simulink model "final_project"  (R2022a)
settings: Solver=VariableStepAuto  StartTime=0.0  StopTime=12  RelTol=1e-3
undefined symbols (not defined in the file or in its folder): C, vinit, Vref
libraries: SignalEditorBlockLib x2
settings Model: Creator=risha  LastModifiedBy=risha

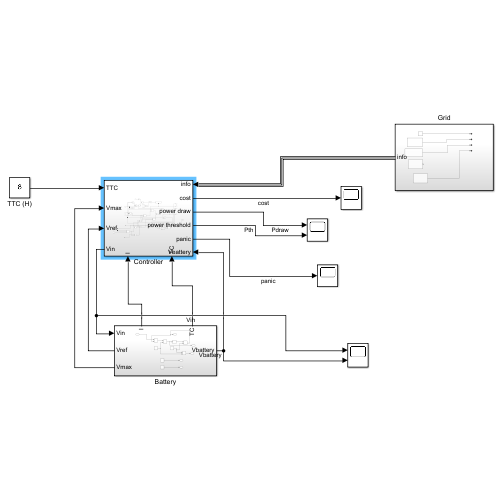
[thumbnail: Simulink's stored preview of the top-level diagram]
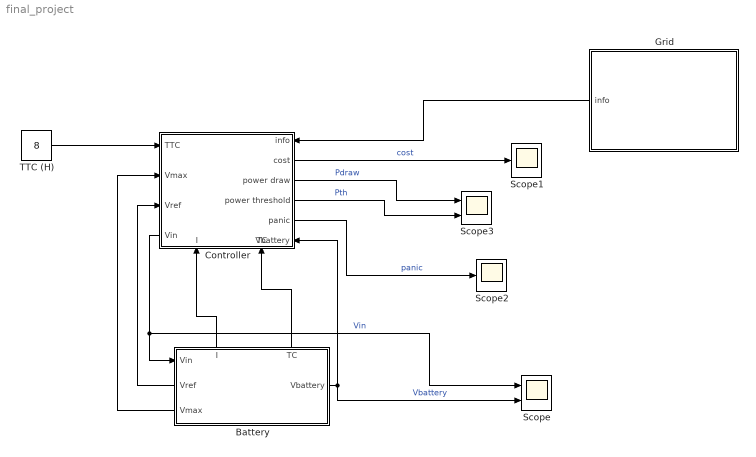
== system final_project ==
  Battery : Subsystem
      settings: PortSchema="{\"entries\":[{\"content\":{\"sides\":[{\"content\":{\"connectorIds\":[\"In1\",\"Out4\",\"Out5\"]},\"type\":\"ConnectorPlacement.EquallySpacedRectSide\",\"uuid\":\"c26d1ca6-d5c6-41a9-a1a0-e3693243df6e\"},{\"content\":{\"connectorIds\":[\"Out1\"],\"side\":\"RIGHT\"},\"type\":\"ConnectorPlacement.EquallySpacedRectSide\",\"uuid\":\"035a91c5-644a-4a3c-8d91-d0006be2b843\"},{\"content\":{\"connectorIds\":[\"Out2\",\"Out3\"],\"side\":\"TOP\"},\"type\":\"ConnectorPlacement.EquallySpacedRectSide\",\"uuid\":\"240e333e-0db7-4e7b-b69e-e92fd9d26be7\"}]},\"type\":\"ConnectorPlacement.EquallySpacedConnector\",\"uuid\":\"79b69b51-48a7-4588-8c16-b604fd62fdea\"}],\"packageUris\":[\"http://schema.mathworks.com/mf0/Connector/R2020b\"],\"version\":\"1.0\"}"
  Controller : Subsystem
      settings: PortSchema="{\"entries\":[{\"content\":{\"sides\":[{\"content\":{\"connectorIds\":[\"In1\",\"In2\",\"In3\",\"Out5\"]},\"type\":\"ConnectorPlacement.EquallySpacedRectSide\",\"uuid\":\"c26d1ca6-d5c6-41a9-a1a0-e3693243df6e\"},{\"content\":{\"connectorIds\":[\"In6\",\"Out1\",\"Out2\",\"Out3\",\"Out4\",\"In7\"],\"side\":\"RIGHT\"},\"type\":\"ConnectorPlacement.EquallySpacedRectSide\",\"uuid\":\"035a91c5-644a-4a3c-8d91-d0006be2b843\"},{\"content\":{\"connectorIds\":[],\"side\":\"TOP\"},\"type\":\"ConnectorPlacement.EquallySpacedRectSide\",\"uuid\":\"240e333e-0db7-4e7b-b69e-e92fd9d26be7\"},{\"content\":{\"connectorIds\":[\"In4\",\"In5\"],\"side\":\"BOTTOM\"},\"type\":\"ConnectorPlacement.EquallySpacedRectSide\",\"uuid\":\"1901438f-64d2-437a-91ec-20947983ea35\"}]},\"type\":\"ConnectorPlacement.EquallySpacedConnector\",\"uuid\":\"79b69b51-48a7-4588-8c16-b604fd62fdea\"}],\"packageUris\":[\"http://schema.mathworks.com/mf0/Connector/R2020b\"],\"version\":\"1.0\"}"
  Grid : Subsystem
  Scope : Scope  NumInputPorts=2
  Scope1 : Scope
  Scope2 : Scope
  Scope3 : Scope  NumInputPorts=2
  TTC (H) : Constant  Value=8
  wires:
  Battery/1(Vbattery) -> Scope/2, Controller/7(Vbattery)  "Vbattery"
  Controller/5(Vin) -> Scope/1, Battery/1(Vin)  "Vin"
  Grid/1(info) -> Controller/6(info)
  TTC (H)/1 -> Controller/1(TTC)
  Battery/4(Vref) -> Controller/3(Vref)
  Controller/1(cost) -> Scope1/1  "cost"
  Battery/3(TC) -> Controller/5(TC)
  Battery/5(Vmax) -> Controller/2(Vmax)
  Battery/2(I) -> Controller/4(I)
  Controller/4(panic) -> Scope2/1  "panic"
  Controller/2(power draw) -> Scope3/1  "Pdraw"
  Controller/3(power threshold) -> Scope3/2  "Pth"

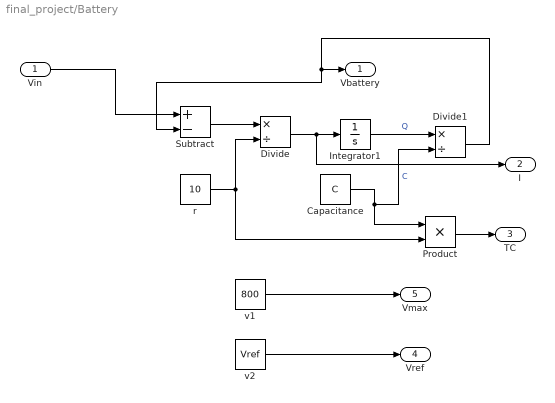
== system final_project/Battery ==
  Vin : Inport
  Capacitance : Constant  Value=C
  Divide : Product  Inputs=*/
  Divide1 : Product  Inputs=*/
  Integrator1 : Integrator  InitialCondition=C*vinit
  Product : Product
  Subtract : Sum  Inputs=+-
  r : Constant  Value=10
  v1 : Constant  Value=800
  v2 : Constant  Value=Vref
  Vbattery : Outport
  I : Outport  Port=2
  TC : Outport  Port=3
  Vref : Outport  Port=4
  Vmax : Outport  Port=5
  wires:
  Vin/1 -> Subtract/1
  Subtract/1 -> Divide/1
  r/1 -> Divide/2, Product/2
  Divide/1 -> I/1, Integrator1/1
  Integrator1/1 -> Divide1/1  "Q"
  Capacitance/1 -> Product/1, Divide1/2  "C"
  Divide1/1 -> Subtract/2, Vbattery/1
  v1/1 -> Vmax/1
  v2/1 -> Vref/1
  Product/1 -> TC/1

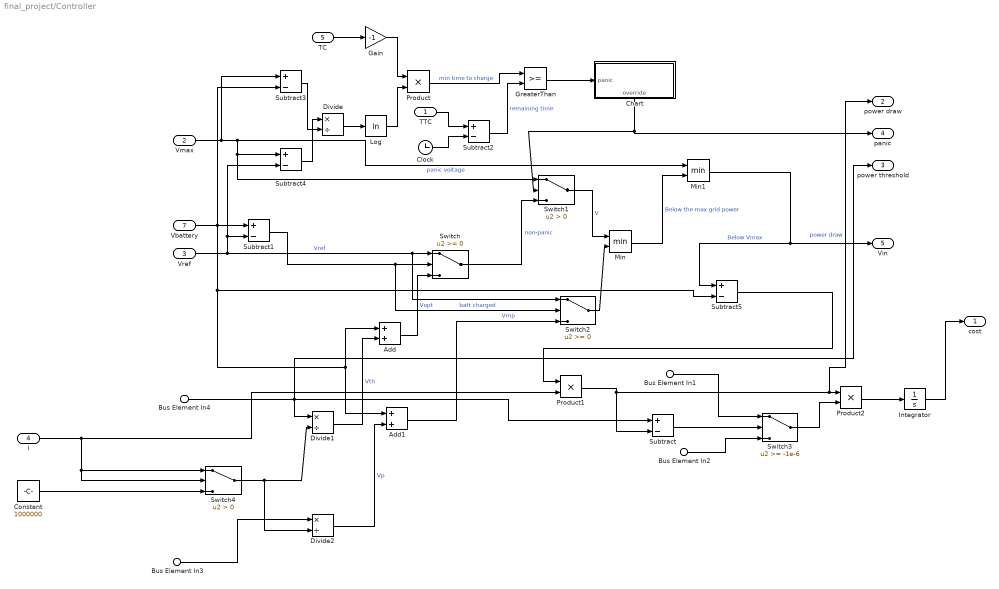
== system final_project/Controller ==
  TTC : Inport
  Vmax : Inport  Port=2
  Vref : Inport  Port=3
  I : Inport  Port=4
  TC : Inport  Port=5
  Bus Element In1 : Inport  Port=6  PortName=info  Element=price1
  Bus Element In3 : Inport  Port=6  PortName=info  Element=max_power
  Bus Element In2 : Inport  Port=6  PortName=info  Element=price2
  Bus Element In4 : Inport  Port=6  PortName=info  Element=threshold
  Vbattery : Inport  Port=7
  Add : Sum
  Add1 : Sum
  Chart : Stateflow chart  TreatAsAtomicUnit=on
      settings: PortSchema="{\"entries\":[{\"content\":{\"sides\":[{\"content\":{\"connectorIds\":[\"In1\"]},\"type\":\"ConnectorPlacement.EquallySpacedRectSide\",\"uuid\":\"c26d1ca6-d5c6-41a9-a1a0-e3693243df6e\"},{\"content\":{\"connectorIds\":[],\"side\":\"RIGHT\"},\"type\":\"ConnectorPlacement.EquallySpacedRectSide\",\"uuid\":\"035a91c5-644a-4a3c-8d91-d0006be2b843\"},{\"content\":{\"connectorIds\":[],\"side\":\"TOP\"},\"type\":\"ConnectorPlacement.EquallySpacedRectSide\",\"uuid\":\"240e333e-0db7-4e7b-b69e-e92fd9d26be7\"},{\"content\":{\"connectorIds\":[\"Out1\"],\"side\":\"BOTTOM\"},\"type\":\"ConnectorPlacement.EquallySpacedRectSide\",\"uuid\":\"c4752108-efdd-4c8c-b1f2-71a131b9b4a8\"}]},\"type\":\"ConnectorPlacement.EquallySpacedConnector\",\"uuid\":\"79b69b51-48a7-4588-8c16-b604fd62fdea\"}],\"packageUris\":[\"http://schema.mathworks.com/mf0/Connector/R2020b\"],\"version\":\"1.0\"}"
  Clock : Clock
  Constant : Constant  Value=1000000
  Divide : Product  Inputs=*/
  Divide1 : Product  Inputs=*/
  Divide2 : Product  Inputs=*/
  Gain : Gain  Gain=-1
  GreaterThan : RelationalOperator  OutDataTypeStr=boolean  RndMeth=Simplest  InputSameDT=off
  Integrator : Integrator
  Log : Math  Operator=log
  Min : MinMax  Inputs=2
  Min1 : MinMax  Inputs=2
  Product : Product
  Product1 : Product
  Product2 : Product
  Subtract{,1..5} (6 alike) : Sum  Inputs=+-
  Switch : Switch  SaturateOnIntegerOverflow=off  InputSameDT=off
  Switch1 : Switch  Criteria=u2 > Threshold  SaturateOnIntegerOverflow=off  InputSameDT=off
  Switch2 : Switch  SaturateOnIntegerOverflow=off  InputSameDT=off
  Switch3 : Switch  Threshold=-1e-6  SaturateOnIntegerOverflow=off  InputSameDT=off
  Switch4 : Switch  Criteria=u2 > Threshold  SaturateOnIntegerOverflow=off  InputSameDT=off
  cost : Outport
  power draw : Outport  Port=2
  power threshold : Outport  Port=3
  panic : Outport  Port=4
  Vin : Outport  Port=5
  wires:
  Chart/1(override) -> panic/1, Switch1/2
  Subtract1/1 -> Switch2/2, Switch/2  "batt charged"
  Vref/1 -> Subtract4/2, Subtract1/2, Switch2/1, Switch/1  "Vref"
  TTC/1 -> Subtract2/1
  Clock/1 -> Subtract2/2
  Subtract2/1 -> GreaterThan/2  "remaining time"
  Vmax/1 -> Subtract3/1, Min1/1, Switch1/1, Subtract4/1  "panic voltage"
  Subtract4/1 -> Divide/1
  Subtract3/1 -> Divide/2
  Divide/1 -> Log/1
  TC/1 -> Gain/1
  Gain/1 -> Product/1
  Log/1 -> Product/2
  Product/1 -> GreaterThan/1  "min time to charge"
  GreaterThan/1 -> Chart/1(panic)
  Switch/1 -> Switch1/3  "non-panic"
  Bus Element In4/1 -> Subtract/1, Divide1/1, power threshold/1
  Divide1/1 -> Add/2  "Vth"
  Add/1 -> Switch/3  "Vopt"
  Bus Element In2/1 -> Switch3/3
  Vbattery/1 -> Add1/1, Add/1, Subtract5/2, Subtract3/2, Subtract1/1
  Bus Element In3/1 -> Divide2/1
  I/1 -> Switch4/2, Switch4/1, Product1/2
  Divide2/1 -> Add1/2  "Vp"
  Switch1/1 -> Min/1  "V"
  Min/1 -> Min1/2  "Below the max grid power"
  Add1/1 -> Switch2/3  "Vmp"
  Switch2/1 -> Min/2
  Subtract/1 -> Switch3/2
  Product1/1 -> Subtract/2, power draw/1, Product2/1  "power draw"
  Bus Element In1/1 -> Switch3/1
  Switch3/1 -> Product2/2
  Product2/1 -> Integrator/1
  Integrator/1 -> cost/1
  Min1/1 -> Subtract5/1, Vin/1  "Below Vmax"
  Constant/1 -> Switch4/3
  Switch4/1 -> Divide2/2, Divide1/2
  Subtract5/1 -> Product1/1

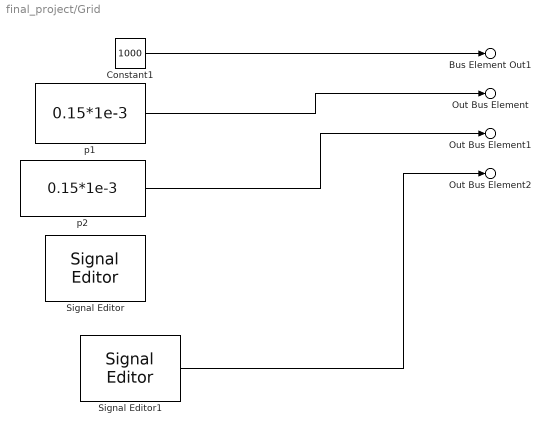
== system final_project/Grid ==
  Constant1 : Constant  Value=1000
  Signal Editor : SignalEditorBlockLib/Signal Editor  FileName=untitled.mat  ActiveScenario=Scenario  ActiveSignal=power_threshold  IsBus=off  OutputBusObjectStr=Bus: BusObject  SampleTime=0  Interpolate=off  ZeroCross=off  OutputAfterFinalValue=Setting to zero  Unit=inherit  PreserveSignalName=on
  Signal Editor1 : SignalEditorBlockLib/Signal Editor  FileName=untitled.mat  ActiveScenario=Scenario  ActiveSignal=power_threshold  IsBus=off  OutputBusObjectStr=Bus: BusObject  SampleTime=0  Interpolate=off  ZeroCross=off  OutputAfterFinalValue=Setting to zero  Unit=inherit  PreserveSignalName=on
  p1 : Constant  Value=0.15*1e-3
  p2 : Constant  Value=0.15*1e-3
  Bus Element Out1 : Outport  PortName=info  Element=max_power
  Out Bus Element : Outport  PortName=info  Element=price1
  Out Bus Element1 : Outport  PortName=info  Element=price2
  Out Bus Element2 : Outport  PortName=info  Element=threshold
  wires:
  Constant1/1 -> Bus Element Out1/1
  p1/1 -> Out Bus Element/1
  p2/1 -> Out Bus Element1/1
  Signal Editor1/1 -> Out Bus Element2/1

== stateflow chart final_project/Controller/Chart ==
  state Optimize
    override=0;
  state Panic
    override=1;
  (default) -> Optimize
  Optimize -> Panic : [panic==1]
  data: panic input; override output
